simulink model "Lift_off_state_test"  (R2017b)
settings: Solver=VariableStepAuto  StartTime=0.0  StopTime=10.0  RelTol=1e-3
settings Model: Creator=Kalana  LastModifiedBy=Kalana

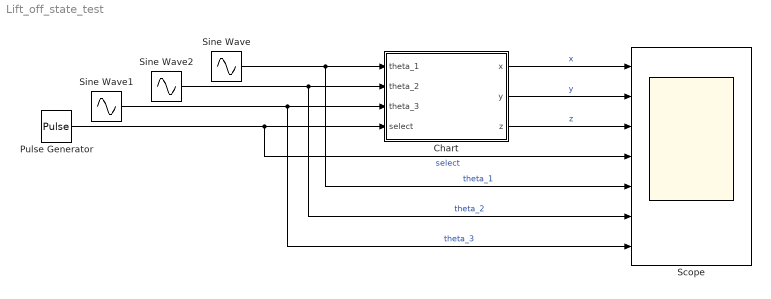
== system Lift_off_state_test ==
  Chart : Stateflow chart  TreatAsAtomicUnit=on
  Pulse Generator : DiscretePulseGenerator  PulseType=Time based  PulseWidth=50  PhaseDelay=-0.6
  Scope : Scope  NumInputPorts=7
  Sine Wave : Sin  Amplitude=0.523  Frequency=0.8  SampleTime=0
  Sine Wave1 : Sin  Amplitude=1.046  Frequency=0.8  SampleTime=0
  Sine Wave2 : Sin  Amplitude=1.04  Frequency=0.8  SampleTime=0
  wires:
  Sine Wave/1 -> Scope/5, Chart/1(theta_1)  "theta_1"
  Sine Wave2/1 -> Scope/6, Chart/2(theta_2)  "theta_2"
  Sine Wave1/1 -> Scope/7, Chart/3(theta_3)  "theta_3"
  Pulse Generator/1 -> Scope/4, Chart/4(select)  "select"
  Chart/1(x) -> Scope/1  "x"
  Chart/2(y) -> Scope/2  "y"
  Chart/3(z) -> Scope/3  "z"

== stateflow chart Lift_off_state_test/Chart ==
  state Set_State_Swing
    entry:x = theta_1
    y = theta_2
    z = theta_3
  state Fixed_State_State
    entry: x = x
    y = y
    z = z
  (default) -> Set_State_Swing
  Set_State_Swing -> Fixed_State_State : [select == 1 ]
  Fixed_State_State -> Set_State_Swing : [select == 0]
  data: theta_1 input; theta_2 input; theta_3 input; select input; x output; y output; z output
